simulink model "P9_TransmisionDigitalEnBandaBase"  (R2020a)
settings: Solver=VariableStepAuto  StartTime=0.0  StopTime=5  FixedStep=1e-5  RelTol=1e-3
libraries: commutil2 x5, commsink2 x2, commfilt2 x2, commchan3 x1, commrandsrc3 x1, dspstat3 x1
settings Model: Creator=León Mora  LastModifiedBy=León Mora

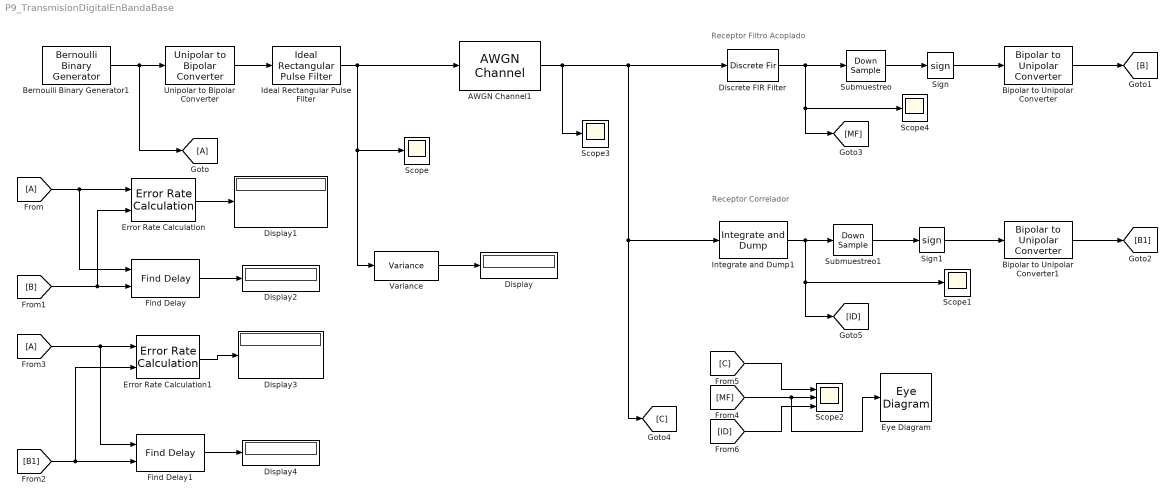
== system P9_TransmisionDigitalEnBandaBase ==
  note: Receptor Correlador
  note: Receptor Filtro Acoplado
  AWGN Channel1 : commchan3/AWGN Channel  InputProcessing=Columns as channels (frame based)  seed=randseed  noiseMode="Signal to noise ratio  (Eb/No)"  EbNodB=3  EsNodB=10  SNRdB=10  bitsPerSym=1  Ps=1  Tsym=1e-3  variance=1
  Bernoulli Binary Generator1 : commrandsrc3/Bernoulli Binary Generator  ProbabilityOfZero=0.5  SeedSource=Auto  Seed=0  SampleTime=0.001  SamplesPerFrame=1  OutputDataType=double  SimulateUsing=Interpreted execution
  Bipolar to Unipolar Converter : commutil2/Bipolar to Unipolar Converter  M=2  polarity=Positive  dataType=Inherit via internal rule
      settings: SourceProductBaseCode=CM
  Bipolar to Unipolar Converter1 : commutil2/Bipolar to Unipolar Converter  M=2  polarity=Positive  dataType=Inherit via internal rule
      settings: SourceProductBaseCode=CM
  Discrete FIR Filter : DiscreteFir  Coefficients=ones(1,100)
  Display{,1..4} (5 alike) : Display
  Error Rate Calculation : commsink2/Error Rate Calculation  N=1  st_delay=0  cp_mode=Entire frame  subframe=[]  PMode=Port  WsName=ErrorVec  RsMode2=off  stop=off  numErr=100  maxBits=1e6
  Error Rate Calculation1 : commsink2/Error Rate Calculation  N=1  st_delay=0  cp_mode=Entire frame  subframe=[]  PMode=Port  WsName=ErrorVec  RsMode2=off  stop=off  numErr=100  maxBits=1e6
  Eye Diagram : EyeDiagram
  Find Delay : commutil2/Find Delay  corrLength=200  chgSigOP=off  stopUpdate=off  numConstDelay=3
      settings: SourceProductBaseCode=CM
  Find Delay1 : commutil2/Find Delay  corrLength=200  chgSigOP=off  stopUpdate=off  numConstDelay=3
      settings: SourceProductBaseCode=CM
  Ideal Rectangular Pulse Filter : commfilt2/Ideal Rectangular Pulse Filter  pulseLen=100  pulseDelay=0  RateOptions=Allow multirate processing  sampMode=Mute  normCheck=off  normMode=Sum of samples  filterGain=1  saveAsFlag=0  roundingMode=Floor  overflowMode=off  firstCoeffDataTypeStr=Inherit: Same word length as input  firstCoeffMin=[]  firstCoeffMax=[]  firstCoeffLastDataTypeStr=Inherit: Same word length as input  outputDataTypeStr=Inherit: Same as accumulator  outputMin=[]  outputMax=[]  outputLastDataTypeStr=Inherit: Same as accumulator
      settings: SourceProductBaseCode=CM
  Integrate and Dump1 : commfilt2/Integrate and Dump  obssamples=100  offsetsamples=0  nodump=on  roundingMode=Floor  overflowMode=off  outputDataTypeStr=Inherit: Same as accumulator  outputLastDataTypeStr=Inherit: Same as accumulator
  Scope{,1,3..4} (4 alike) : Scope
  Scope2 : Scope  NumInputPorts=3
  Sign : Signum
  Sign1 : Signum
  Submuestreo : DownSample  N=100  phase=99  RateOptions=Allow multirate processing
  Submuestreo1 : DownSample  N=100  phase=99  RateOptions=Allow multirate processing
  Unipolar to Bipolar Converter : commutil2/Unipolar to Bipolar Converter  M=2  polarity=Positive  dataType=Inherit via internal rule
  Variance : dspstat3/Variance  run=on  reset_popup=None  directionMode=Each column  dimension=1  roiEnable=off  roiType=Rectangles  roiPortion=Entire ROI  roiOutput=Individual statistics for each ROI  roiFlag=off  roundingMode=Floor  overflowMode=off
  wires:
  Bernoulli Binary Generator1/1 -> [A], Unipolar to Bipolar Converter/1
  Unipolar to Bipolar Converter/1 -> Ideal Rectangular Pulse Filter/1
  Ideal Rectangular Pulse Filter/1 -> AWGN Channel1/1, Variance/1, Scope/1
  Variance/1 -> Display/1
  Discrete FIR Filter/1 -> [MF], Scope4/1, Submuestreo/1
  Submuestreo/1 -> Sign/1
  Sign/1 -> Bipolar to Unipolar Converter/1
  AWGN Channel1/1 -> [C], Integrate and Dump1/1, Discrete FIR Filter/1, Scope3/1
  Integrate and Dump1/1 -> [ID], Scope1/1, Submuestreo1/1
  Submuestreo1/1 -> Sign1/1
  Sign1/1 -> Bipolar to Unipolar Converter1/1
  [A] -> Find Delay/1, Error Rate Calculation/1
  Bipolar to Unipolar Converter/1 -> [B]
  [B] -> Error Rate Calculation/2, Find Delay/2
  Bipolar to Unipolar Converter1/1 -> [B1]
  Error Rate Calculation/1 -> Display1/1
  Find Delay/1 -> Display2/1
  [A] -> Find Delay1/1, Error Rate Calculation1/1
  Error Rate Calculation1/1 -> Display3/1
  [B1] -> Find Delay1/2, Error Rate Calculation1/2
  Find Delay1/1 -> Display4/1
  [C] -> Scope2/1
  [ID] -> Scope2/3
  [MF] -> Eye Diagram/1, Scope2/2
